simulink model "PID_S_Shape_Tuning"  (R2023a)
settings: Solver=VariableStepAuto  StartTime=0.0  StopTime=20  MaxStep=0.001  RelTol=1e-3
libraries: simulink x1
settings Model: Creator=Mohamed Ezzelrgal  LastModifiedBy=Mohamed Ezzelrgal

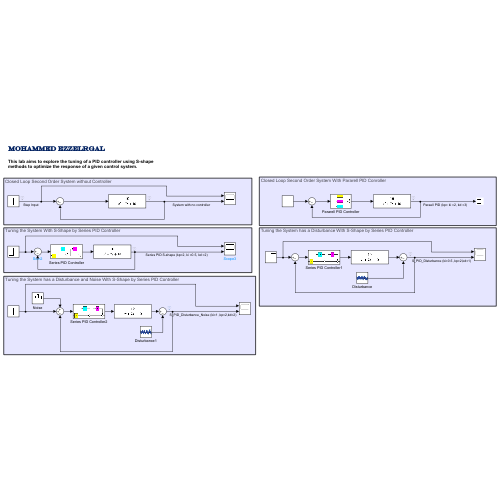
[thumbnail: Simulink's stored preview of the top-level diagram]
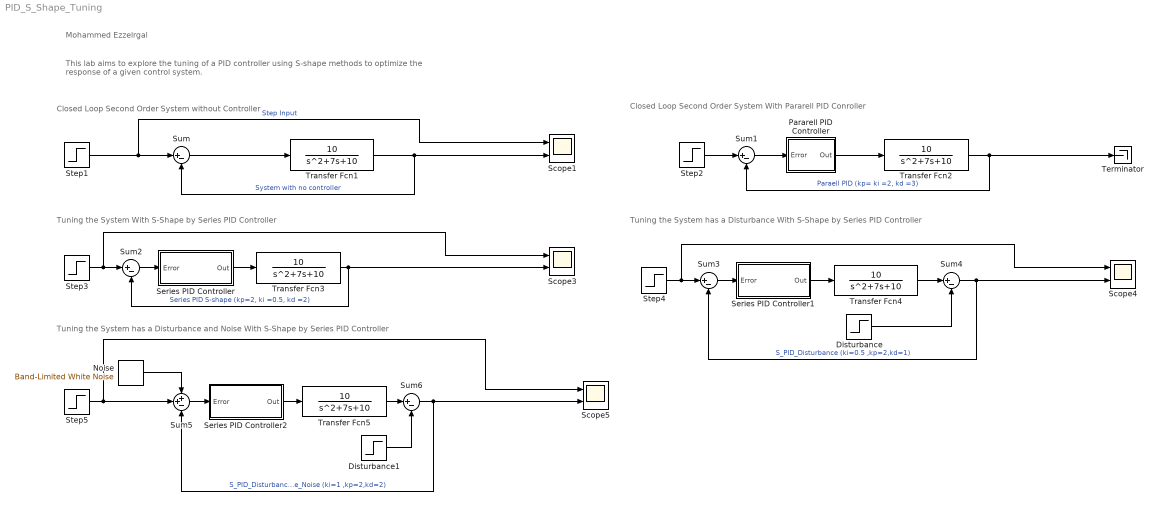
== system PID_S_Shape_Tuning ==
  note: Tuning the System With S-Shape by Series PID Controller
  note: Closed Loop Second Order System With Pararell PID Conroller
  note: Closed Loop Second Order System without Controller
  note: This lab aims to explore the tuning of a PID controller using S-shape methods to optimize the response of a given control system.
  note: Mohammed Ezzelrgal
  note: Tuning the System has a Disturbance With S-Shape by Series PID Controller
  note: Tuning the System has a Disturbance and Noise With S-Shape by Series PID Controller
  Disturbance : Step  Time=5  After=0.5  SampleTime=0
      mask Display: image('C:\Users\User\Pictures\Screenshots\Screenshot 2024-04-04 034433.png'); % Use "Edit Image" on toolstrip to change.
  Disturbance1 : Step  Time=20  After=0.5  SampleTime=0
      mask Display: image('C:\Users\User\Pictures\Screenshots\Screenshot 2024-04-04 034433.png'); % Use "Edit Image" on toolstrip to change.
  Noise : simulink/Sources/Band-Limited White Noise  Cov=[0.000001]  Ts=0.2  seed=[23341]
  Pararell PID Controller : Subsystem
      mask Display: image('C:\Users\User\Pictures\Screenshots\Screenshot 2024-04-04 033959.png'); % Use "Edit Image" on toolstrip to change.
  Scope{1,3..5} (4 alike) : Scope  NumInputPorts=2
  Series PID Controller : Subsystem
      mask Display: image('C:\Users\User\Pictures\Screenshots\Screenshot 2024-04-04 033454.png'); % Use "Edit Image" on toolstrip to change.
  Series PID Controller1 : Subsystem
      mask Display: image('C:\Users\User\Pictures\Screenshots\Screenshot 2024-04-04 033454.png'); % Use "Edit Image" on toolstrip to change.
  Series PID Controller2 : Subsystem
      mask Display: image('C:\Users\User\Pictures\Screenshots\Screenshot 2024-04-04 033454.png'); % Use "Edit Image" on toolstrip to change.
  Step{1..5} (5 alike) : Step  SampleTime=0
  Sum{,1..4,6} (6 alike) : Sum  Inputs=|+-
  Sum5 : Sum  Inputs=++-
  Terminator : Terminator
  Transfer Fcn{1..5} (5 alike) : TransferFcn  Numerator=[10]  Denominator=[1 7 10]
  wires:
  Transfer Fcn1/1 -> Scope1/2, Sum/2  "System with no controller"
  Sum/1 -> Transfer Fcn1/1
  Step1/1 -> Scope1/1, Sum/1  "Step Input"
  Step2/1 -> Sum1/1
  Transfer Fcn2/1 -> Sum1/2, Terminator/1  "Paraell PID (kp= ki =2, kd =3)"
  Pararell PID Controller/1(Out) -> Transfer Fcn2/1
  Sum1/1 -> Pararell PID Controller/1(Error)
  Sum2/1 -> Series PID Controller/1(Error)
  Series PID Controller/1(Out) -> Transfer Fcn3/1
  Transfer Fcn3/1 -> Scope3/2, Sum2/2  "Series PID S-shape (kp=2, ki =0.5, kd =2)"
  Step3/1 -> Sum2/1, Scope3/1
  Step4/1 -> Scope4/1, Sum3/1
  Series PID Controller1/1(Out) -> Transfer Fcn4/1
  Sum3/1 -> Series PID Controller1/1(Error)
  Disturbance/1 -> Sum4/2
  Transfer Fcn4/1 -> Sum4/1
  Sum4/1 -> Sum3/2, Scope4/2  "S_PID_Disturbance (ki=0.5 ,kp=2,kd=1)"
  Sum6/1 -> Scope5/2, Sum5/3  "S_PID_Disturbance_Noise (ki=1 ,kp=2,kd=2)"
  Transfer Fcn5/1 -> Sum6/1
  Disturbance1/1 -> Sum6/2
  Sum5/1 -> Series PID Controller2/1(Error)
  Series PID Controller2/1(Out) -> Transfer Fcn5/1
  Step5/1 -> Scope5/1, Sum5/2
  Noise/1 -> Sum5/1

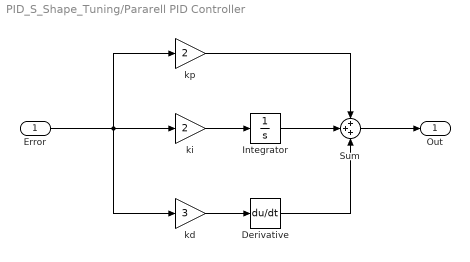
== system PID_S_Shape_Tuning/Pararell PID Controller ==
  Error : Inport
  Derivative : Derivative
  Integrator : Integrator
  Sum : Sum  Inputs=+++
  kd : Gain  Gain=3
  ki : Gain  Gain=2
  kp : Gain  Gain=2
  Out : Outport
  wires:
  ki/1 -> Integrator/1
  kd/1 -> Derivative/1
  Integrator/1 -> Sum/2
  kp/1 -> Sum/1
  Derivative/1 -> Sum/3
  Error/1 -> kd/1, kp/1, ki/1
  Sum/1 -> Out/1

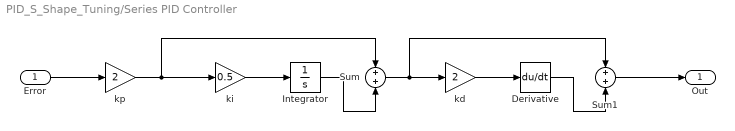
== system PID_S_Shape_Tuning/Series PID Controller ==
  Error : Inport
  Derivative : Derivative
  Integrator : Integrator
  Sum : Sum
  Sum1 : Sum
  kd : Gain  Gain=2
  ki : Gain  Gain=0.5
  kp : Gain  Gain=2
  Out : Outport
  wires:
  Error/1 -> kp/1
  kd/1 -> Derivative/1
  ki/1 -> Integrator/1
  kp/1 -> Sum/1, ki/1
  Integrator/1 -> Sum/2
  Sum1/1 -> Out/1
  Sum/1 -> Sum1/1, kd/1
  Derivative/1 -> Sum1/2

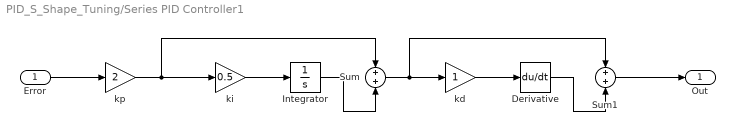
== system PID_S_Shape_Tuning/Series PID Controller1 ==
  Error : Inport
  Derivative : Derivative
  Integrator : Integrator
  Sum : Sum
  Sum1 : Sum
  kd : Gain
  ki : Gain  Gain=0.5
  kp : Gain  Gain=2
  Out : Outport
  wires:
  Derivative/1 -> Sum1/2
  Sum/1 -> kd/1, Sum1/1
  Sum1/1 -> Out/1
  Integrator/1 -> Sum/2
  kp/1 -> ki/1, Sum/1
  ki/1 -> Integrator/1
  kd/1 -> Derivative/1
  Error/1 -> kp/1

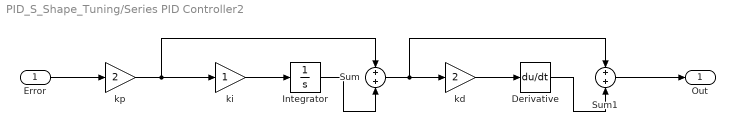
== system PID_S_Shape_Tuning/Series PID Controller2 ==
  Error : Inport
  Derivative : Derivative
  Integrator : Integrator
  Sum : Sum
  Sum1 : Sum
  kd : Gain  Gain=2
  ki : Gain
  kp : Gain  Gain=2
  Out : Outport
  wires:
  Error/1 -> kp/1
  kd/1 -> Derivative/1
  ki/1 -> Integrator/1
  kp/1 -> Sum/1, ki/1
  Integrator/1 -> Sum/2
  Sum1/1 -> Out/1
  Sum/1 -> Sum1/1, kd/1
  Derivative/1 -> Sum1/2
